simulink model "lab02"  (R2020b)
settings: Solver=VariableStepAuto  StartTime=0.0  StopTime=10.0  RelTol=1e-3
model workspace (MAT data in the model file):
  Fn = Simulink.Parameter
  Fn.Value = 1
  Fn.DataType = 'auto'
  Fn.Dimensions = [1 1]
  Tin = Simulink.Parameter
  Tin.Value = 1
  Tin.DataType = 'auto'
  Tin.Dimensions = [1 1]
undefined symbols (not defined in the file): be, bv, le, lv, muk, mus, R
settings Model: Creator=karth  LastModifiedBy=karth

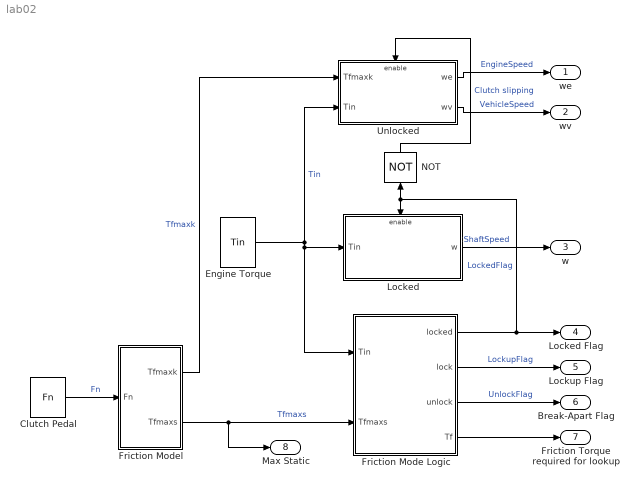
== system lab02 ==
  " Clutch Pedal" : FromWorkspace  VariableName=Fn  SampleTime=1  ZeroCross=off
  Engine Torque : FromWorkspace  VariableName=Tin  ZeroCross=off
  Friction Mode Logic : Subsystem
  Friction Model : Subsystem
  Locked : Subsystem
  NOT : Logic  Operator=NOT  IconShape=distinctive  AllPortsSameDT=off  OutDataTypeStr=boolean
  Unlocked : Subsystem
  we : Outport
  wv : Outport  Port=2
  w : Outport  Port=3
  Locked Flag : Outport  Port=4
  Lockup Flag : Outport  Port=5
  Break-Apart Flag : Outport  Port=6
  Friction Torque required for lookup : Outport  Port=7
  Max Static : Outport  Port=8
  wires:
  Friction Mode Logic/4(Tf) -> Friction Torque required for lookup/1
  Friction Mode Logic/3(unlock) -> Break-Apart Flag/1  "UnlockFlag"
  Unlocked/2(wv) -> wv/1  "VehicleSpeed"
  Friction Model/1(Tfmaxk) -> Unlocked/1(Tfmaxk)  "Tfmaxk"
  Friction Model/2(Tfmaxs) -> Max Static/1, Friction Mode Logic/2(Tfmaxs)  "Tfmaxs"
  Friction Mode Logic/2(lock) -> Lockup Flag/1  "LockupFlag"
  Engine Torque/1 -> Locked/1(Tin), Friction Mode Logic/1(Tin), Unlocked/2(Tin)  "Tin"
  NOT/1 -> Unlocked/Enable  "Clutch slipping"
  Unlocked/1(we) -> we/1  "EngineSpeed"
  " Clutch Pedal"/1 -> Friction Model/1(Fn)  "Fn"
  Locked/1(w) -> w/1  "ShaftSpeed"
  Friction Mode Logic/1(locked) -> Locked Flag/1, Locked/Enable, NOT/1  "LockedFlag"

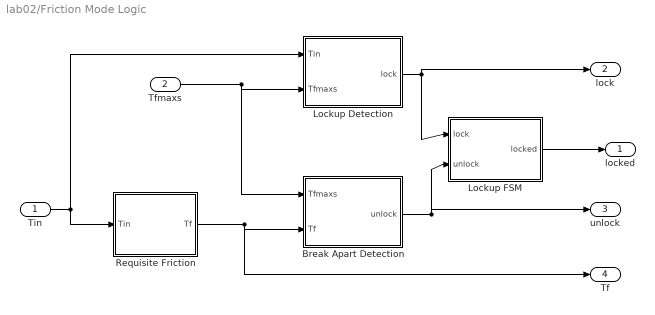
== system lab02/Friction Mode Logic ==
  Tin : Inport
  Tfmaxs : Inport  Port=2
  Break Apart Detection : Subsystem
  Lockup Detection : Subsystem
  Lockup FSM : Subsystem
  Requisite Friction : Subsystem
  locked : Outport
  lock : Outport  Port=2
  unlock : Outport  Port=3
  Tf : Outport  Port=4
  wires:
  Break Apart Detection/1(unlock) -> unlock/1, Lockup FSM/2(unlock)
  Tfmaxs/1 -> Break Apart Detection/1(Tfmaxs), Lockup Detection/2(Tfmaxs)
  Lockup Detection/1(lock) -> lock/1, Lockup FSM/1(lock)
  Tin/1 -> Lockup Detection/1(Tin), Requisite Friction/1(Tin)
  Requisite Friction/1(Tf) -> Tf/1, Break Apart Detection/2(Tf)
  Lockup FSM/1(locked) -> locked/1

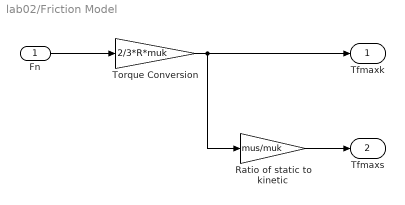
== system lab02/Friction Model ==
  Fn : Inport
  Ratio of static to kinetic : Gain  Gain=mus/muk
  Torque Conversion : Gain  Gain=2/3*R*muk
  Tfmaxk : Outport
  Tfmaxs : Outport  Port=2
  wires:
  Torque Conversion/1 -> Tfmaxk/1, Ratio of static to kinetic/1
  Fn/1 -> Torque Conversion/1
  Ratio of static to kinetic/1 -> Tfmaxs/1

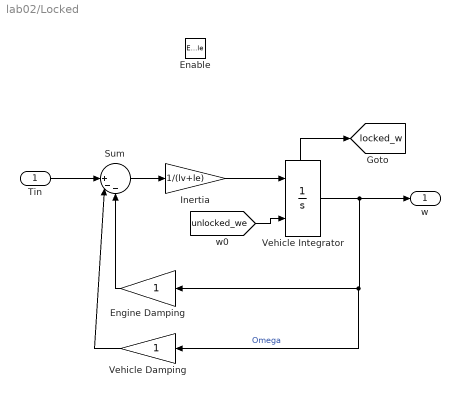
== system lab02/Locked ==
  Tin : Inport
  Enable : EnablePort
  Engine Damping : Gain
  Inertia : Gain  Gain=1/(lv+le)
  Sum : Sum  Inputs=||+--
  Vehicle Damping : Gain
  Vehicle Integrator : Integrator  InitialConditionSource=external  ShowStatePort=on
  w : Outport
  tag scope: locked_w=global
  wires:
  Inertia/1 -> Vehicle Integrator/1
  Vehicle Integrator/1 -> w/1, Vehicle Damping/1, Engine Damping/1  "Omega"
  Tin/1 -> Sum/1
  Vehicle Integrator/State -> [locked_w]
  Sum/1 -> Inertia/1
  Vehicle Damping/1 -> Sum/2
  [unlocked_we] -> Vehicle Integrator/2
  Engine Damping/1 -> Sum/3

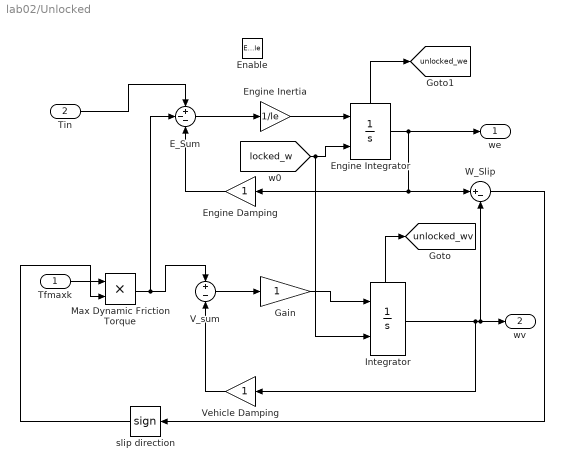
== system lab02/Unlocked ==
  Tfmaxk : Inport
  Tin : Inport  Port=2
  Enable : EnablePort
  E_Sum : Sum  Inputs=+--
  Engine Damping : Gain
  Engine Inertia : Gain  Gain=1/le
  Engine Integrator : Integrator  InitialConditionSource=external  ShowStatePort=on
  Gain : Gain
  Integrator : Integrator  InitialConditionSource=external  ShowStatePort=on
  Max Dynamic Friction Torque : Product
  V_sum : Sum  Inputs=+-
  Vehicle Damping : Gain
  W_Slip : Sum  Inputs=|+-  InputSameDT=on  SaturateOnIntegerOverflow=on  OutDataTypeStr=Inherit: Same as first input
  slip direction : Signum
  we : Outport
  wv : Outport  Port=2
  tag scope: unlocked_we=global, unlocked_wv=global
  wires:
  slip direction/1 -> Max Dynamic Friction Torque/2
  Integrator/1 -> wv/1, W_Slip/2, Vehicle Damping/1
  Tin/1 -> E_Sum/1
  Engine Damping/1 -> E_Sum/3
  Gain/1 -> Integrator/1
  Engine Integrator/1 -> we/1, Engine Damping/1, W_Slip/1
  Max Dynamic Friction Torque/1 -> E_Sum/2, V_sum/1
  Engine Integrator/State -> [unlocked_we]
  E_Sum/1 -> Engine Inertia/1
  W_Slip/1 -> slip direction/1
  V_sum/1 -> Gain/1
  Tfmaxk/1 -> Max Dynamic Friction Torque/1
  Vehicle Damping/1 -> V_sum/2
  Engine Inertia/1 -> Engine Integrator/1
  Integrator/State -> [unlocked_wv]
  [locked_w] -> Integrator/2, Engine Integrator/2

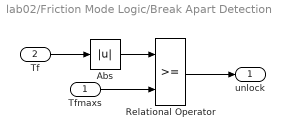
== system lab02/Friction Mode Logic/Break Apart Detection ==
  Tfmaxs : Inport
  Tf : Inport  Port=2
  Abs : Abs
  Relational Operator : RelationalOperator  OutDataTypeStr=boolean  RndMeth=Simplest
  unlock : Outport
  wires:
  Tf/1 -> Abs/1
  Relational Operator/1 -> unlock/1
  Tfmaxs/1 -> Relational Operator/2
  Abs/1 -> Relational Operator/1

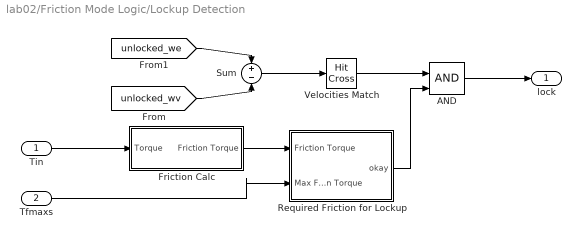
== system lab02/Friction Mode Logic/Lockup Detection ==
  Tin : Inport
  Tfmaxs : Inport  Port=2
  AND : Logic  IconShape=distinctive  AllPortsSameDT=off  OutDataTypeStr=boolean
  Friction Calc : Subsystem
  Required Friction for Lockup : Subsystem
  Sum : Sum  Inputs=+-
  Velocities Match : HitCross
  lock : Outport
  wires:
  [unlocked_wv] -> Sum/2
  Velocities Match/1 -> AND/1
  AND/1 -> lock/1
  Tin/1 -> Friction Calc/1(Torque)
  Required Friction for Lockup/1(okay) -> AND/2
  Friction Calc/1(Friction Torque) -> Required Friction for Lockup/1(Friction Torque)
  [unlocked_we] -> Sum/1
  Sum/1 -> Velocities Match/1
  Tfmaxs/1 -> Required Friction for Lockup/2(Max Friction Torque)

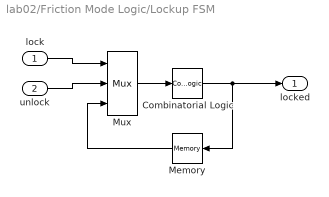
== system lab02/Friction Mode Logic/Lockup FSM ==
  lock : Inport
  unlock : Inport  Port=2
  Combinatorial Logic : CombinatorialLogic  TruthTable=[0;1;0;0;1;1;1;0]
  Memory : Memory
  Mux : Mux  Inputs=3
  locked : Outport  InitialOutput=0  VectorParamsAs1DForOutWhenUnconnected=off
  wires:
  Mux/1 -> Combinatorial Logic/1
  lock/1 -> Mux/1
  unlock/1 -> Mux/2
  Combinatorial Logic/1 -> locked/1, Memory/1
  Memory/1 -> Mux/3

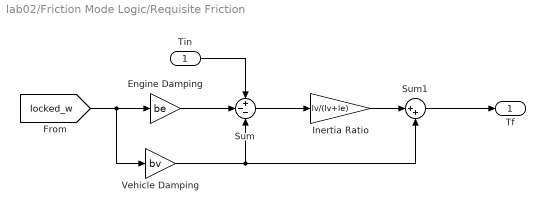
== system lab02/Friction Mode Logic/Requisite Friction ==
  Tin : Inport
  Engine Damping : Gain  Gain=be
  Inertia Ratio : Gain  Gain=lv/(lv+le)
  Sum : Sum  Inputs=+--
  Sum1 : Sum  Inputs=|++
  Vehicle Damping : Gain  Gain=bv
  Tf : Outport
  wires:
  [locked_w] -> Vehicle Damping/1, Engine Damping/1
  Engine Damping/1 -> Sum/2
  Sum1/1 -> Tf/1
  Inertia Ratio/1 -> Sum1/1
  Sum/1 -> Inertia Ratio/1
  Vehicle Damping/1 -> Sum1/2, Sum/3
  Tin/1 -> Sum/1

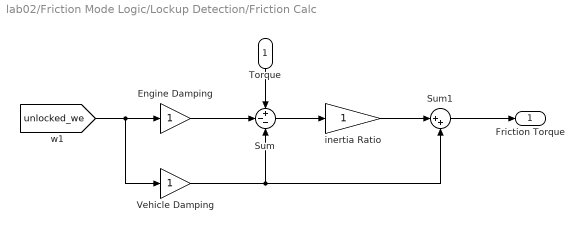
== system lab02/Friction Mode Logic/Lockup Detection/Friction Calc ==
  Torque : Inport
  Engine Damping : Gain
  Sum : Sum  Inputs=+--
  Sum1 : Sum  Inputs=|++
  Vehicle Damping : Gain
  inertia Ratio : Gain
  Friction Torque : Outport
  wires:
  Sum1/1 -> Friction Torque/1
  inertia Ratio/1 -> Sum1/1
  Engine Damping/1 -> Sum/2
  Torque/1 -> Sum/1
  Vehicle Damping/1 -> Sum1/2, Sum/3
  [unlocked_we] -> Vehicle Damping/1, Engine Damping/1
  Sum/1 -> inertia Ratio/1

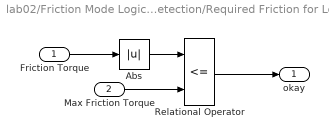
== system lab02/Friction Mode Logic/Lockup Detection/Required Friction for Lockup ==
  Friction Torque : Inport
  Max Friction Torque : Inport  Port=2
  Abs : Abs
  Relational Operator : RelationalOperator  Operator=<=  OutDataTypeStr=boolean  RndMeth=Simplest
  okay : Outport
  wires:
  Max Friction Torque/1 -> Relational Operator/2
  Abs/1 -> Relational Operator/1
  Relational Operator/1 -> okay/1
  Friction Torque/1 -> Abs/1
